simulink model "DemonstratorSimscape"  (R2020b)
settings: Solver=ode113  StartTime=0.0  StopTime=t_stop*0+20  FixedStep=1e-4
values from neighbouring files (symbols this model uses):
  brkD = 0    [main.m]
  brkI = 1e4    (= 10000)    [main.m]
  brkP = 1e5    (= 100000)    [main.m]
  d_drm = 0.5*d_drum    [main.m]
  d_shm = 0.4*d_sheave    [main.m]
  DeltaCable0 = 0    [main.m]
  Droop_scaling = 0    [main.m]
  eta_sh = 0.015    [main.m]
  filt_NUM = ones(1,200)*0.005    [main.m]
  g = 9.80665    [main.m]
  Iw = 0.5*(W.i + M.in*GB.r^2)    [main.m]
  Kp_mul = 0.3    [main.m]
  Lc0 = abs((T.ph-L.height-P.d-L.z0)*0.001)    [main.m]
  Ls1 = ((T.ph-0.5*W.pd)/1000)    [main.m]
  Ls2 = ((0.5*(T.s2+P.d)-2*P.d)/1000)    [main.m]
  M = 50e3    (= 50000)    [calcGrav.m]
  phi0_drm = -90    [main.m]
  phi0_shm = -90    [main.m]
  r_sheave = P.d*0.5    [main.m]
  s = tf('s')    [calcGrav.m]
  tau_brk = 0.001    [main.m]
  tau_em = 60e-3    (= 0.06)    [calcGrav.m]    (also in main.m)
  tau_m = tau_w/GB.r    [main.m]
  Tmax = 400e3    (= 400000)    [main.m]
  Tn_mul = 10    [main.m]
  x_drm = 0.7*r_drum    [main.m]
  x_shm = 0.7*r_sheave    [main.m]
  z0 = 0    [calcGrav.m]    (also in main.m = L.z0-P.d*0.5-P.d-P.d-L.height-T.h1-T.h2-32)
undefined symbols (not defined in the file or in its folder): C, CA, Controller_sampleTime, DiscIntNeverNeededParam, GB, L, P, Part, T, VFD_acceleration_model_factor, VFD_Adapt_factor_lower_p1458, VFD_Adapt_factor_upper_p1459, VFD_Curr_limit_var_p0641, VFD_Current_limit_p0640, VFD_Id_setp_total_r1624, VFD_Iq, VFD_Kp_n_basic_p1460, VFD_M, VFD_M_accel_T_smooth_p1517, VFD_M_lim_var_fixS_src_p1551, VFD_M_max_lower_p1521, VFD_M_max_lower_scal_p1525, VFD_M_max_up_mot_scal_p1524, VFD_M_max_upper_p1520, VFD_n_act_T_smooth_p1442, VFD_n_ctr_Kp_n_up_scal_p1461, VFD_n_ctr_Tn_n_up_sca_p1463, VFD_n_ctrl_adapt_Kp_lower_p1456, VFD_n_ctrl_adapt_Kp_upper_p1457, VFD_n_ctrl_Adpt_sig_Kp_p1455, VFD_n_ctrl_Kp_scal_p1466, VFD_n_ctrl_n_lower_p1464, VFD_n_ctrl_n_upper_p1465, VFD_n_ctrl_Tn_n_lower_p1462, VFD_n_limit_neg_p1086, VFD_n_limit_pos_p1083, VFD_n_limit_setp_p1063, VFD_n_max_p1082, VFD_n_set_filt_1_T_p1416, VFD_P_max_gen_p1531, VFD_P_max_mot_p1530, VFD_PU_I_outp_max_r0289, VFD_RFG_ramp_down_time_p1121, VFD_RFG_ramp_up_time_p1120, VFD_RFG_t_RD_scal_p1139, VFD_RFG_t_RU_scal_p1138, VSD, W, X, Y, Z
libraries: sm_lib x248, nesl_utility x128, simulink x49, pid_lib x4, cstblocks x2, simulink_extras x2
(part 8 of 10)

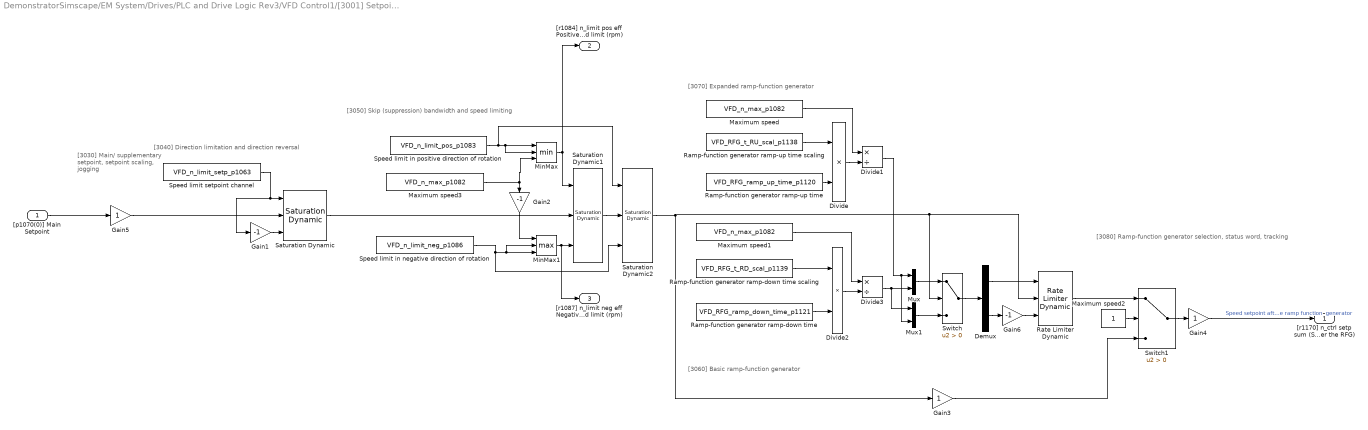
== system DemonstratorSimscape/EM System/Drives/PLC and Drive Logic Rev3/VFD Control1/[3001] Setpoint Channel  ==
  note: [3080] Ramp-function generator selection,
      | status word, tracking
  note: [3070] Expanded ramp-function generator
  note: [3040] Direction limitation and direction reversal
  note: [3050] Skip (suppression) bandwidth
      |  and speed limiting
  note: [3060] Basic ramp-function generator
  note: [3030] Main/
      | supplementary
      | setpoint,
      | setpoint
      | scaling,
      | jogging
  "[p1070(0)] Main Setpoint" : Inport
  Demux : Demux  Outputs=2
  Divide : Product  Inputs=**
  Divide1 : Product  Inputs=*/
  Divide2 : Product  Inputs=**
  Divide3 : Product  Inputs=*/
  Gain1 : Gain  Gain=-1
  Gain2 : Gain  Gain=-1
  Gain3 : Gain
  Gain4 : Gain
  Gain5 : Gain
  Gain6 : Gain  Gain=-1
  Maximum speed : Constant  Value=VFD_n_max_p1082
  Maximum speed1 : Constant  Value=VFD_n_max_p1082
  Maximum speed2 : Constant
  Maximum speed3 : Constant  Value=VFD_n_max_p1082
  MinMax : MinMax  Inputs=3
  MinMax1 : MinMax  Function=max  Inputs=3
  Mux : Mux  Inputs=2
  Mux1 : Mux  Inputs=2
  Ramp-function generator ramp-down time : Constant  Value=VFD_RFG_ramp_down_time_p1121
  Ramp-function generator ramp-down time scaling : Constant  Value=VFD_RFG_t_RD_scal_p1139  VectorParams1D=off
  "Ramp-function generator ramp-up time " : Constant  Value=VFD_RFG_ramp_up_time_p1120
  "Ramp-function generator ramp-up time scaling " : Constant  Value=VFD_RFG_t_RU_scal_p1138
  Rate Limiter Dynamic : simulink/Discontinuities/Rate Limiter Dynamic
  Saturation Dynamic : simulink/Discontinuities/Saturation Dynamic  OutMin=[]  OutMax=[]  OutDataTypeStr=Inherit: Same as second input  OutDataType=fixdt(1, 16)  OutScaling=2^-10  DoSatur=off
  Saturation Dynamic1 : simulink/Discontinuities/Saturation Dynamic  OutMin=[]  OutMax=[]  OutDataTypeStr=Inherit: Same as second input  OutDataType=fixdt(1, 16)  OutScaling=2^-10  DoSatur=off
  Saturation Dynamic2 : simulink/Discontinuities/Saturation Dynamic  OutMin=[]  OutMax=[]  OutDataTypeStr=Inherit: Same as second input  OutDataType=fixdt(1, 16)  OutScaling=2^-10  DoSatur=off
  "Speed limit in negative direction of rotation " : Constant  Value=VFD_n_limit_neg_p1086
  Speed limit in positive direction of rotation : Constant  Value=VFD_n_limit_pos_p1083
  Speed limit setpoint channel : Constant  Value=VFD_n_limit_setp_p1063
  Switch : Switch  Criteria=u2 > Threshold
  Switch1 : Switch  Criteria=u2 > Threshold
  "[r1170] n_ctrl setp sum (Speed setpoint after the RFG)" : Outport  VectorParamsAs1DForOutWhenUnconnected=off
  "[r1084] n_limit pos eff Positive Speed limit (rpm)" : Outport  Port=2  VectorParamsAs1DForOutWhenUnconnected=off
  "[r1087] n_limit neg eff Negative Speed limit (rpm)" : Outport  Port=3  VectorParamsAs1DForOutWhenUnconnected=off
  wires:
  Speed limit setpoint channel/1 -> Saturation Dynamic/1, Gain1/1
  Gain1/1 -> Saturation Dynamic/3
  "[p1070(0)] Main Setpoint"/1 -> Gain5/1
  MinMax1/1 -> "[r1087] n_limit neg eff Negative Speed limit (rpm)"/1, Saturation Dynamic1/3
  Saturation Dynamic/1 -> Saturation Dynamic1/2
  Speed limit in positive direction of rotation/1 -> Saturation Dynamic2/1, MinMax/2, MinMax/1
  "Speed limit in negative direction of rotation "/1 -> Saturation Dynamic2/3, MinMax1/2, MinMax1/3
  Maximum speed3/1 -> Gain2/1, MinMax/3
  MinMax/1 -> "[r1084] n_limit pos eff Positive Speed limit (rpm)"/1, Saturation Dynamic1/1
  Saturation Dynamic2/1 -> Gain3/1, Rate Limiter Dynamic/2, Switch/2
  Mux/1 -> Switch/1
  Maximum speed/1 -> Divide1/1
  Demux/2 -> Gain6/1
  Divide3/1 -> Mux1/1, Mux/2
  "Ramp-function generator ramp-up time scaling "/1 -> Divide/1
  Mux1/1 -> Switch/3
  Switch/1 -> Demux/1
  Divide1/1 -> Mux/1, Mux1/2
  "Ramp-function generator ramp-up time "/1 -> Divide/2
  Divide2/1 -> Divide3/2
  Maximum speed1/1 -> Divide3/1
  Ramp-function generator ramp-down time scaling/1 -> Divide2/1
  Ramp-function generator ramp-down time/1 -> Divide2/2
  Divide/1 -> Divide1/2
  Demux/1 -> Rate Limiter Dynamic/1
  Gain4/1 -> "[r1170] n_ctrl setp sum (Speed setpoint after the RFG)"/1  "Speed setpoint after  the ramp function  generator"
  Rate Limiter Dynamic/1 -> Switch1/1
  Switch1/1 -> Gain4/1
  Gain3/1 -> Switch1/3
  Maximum speed2/1 -> Switch1/2
  Gain5/1 -> Saturation Dynamic/2
  Gain6/1 -> Rate Limiter Dynamic/3
  Saturation Dynamic1/1 -> Saturation Dynamic2/2
  Gain2/1 -> MinMax1/1

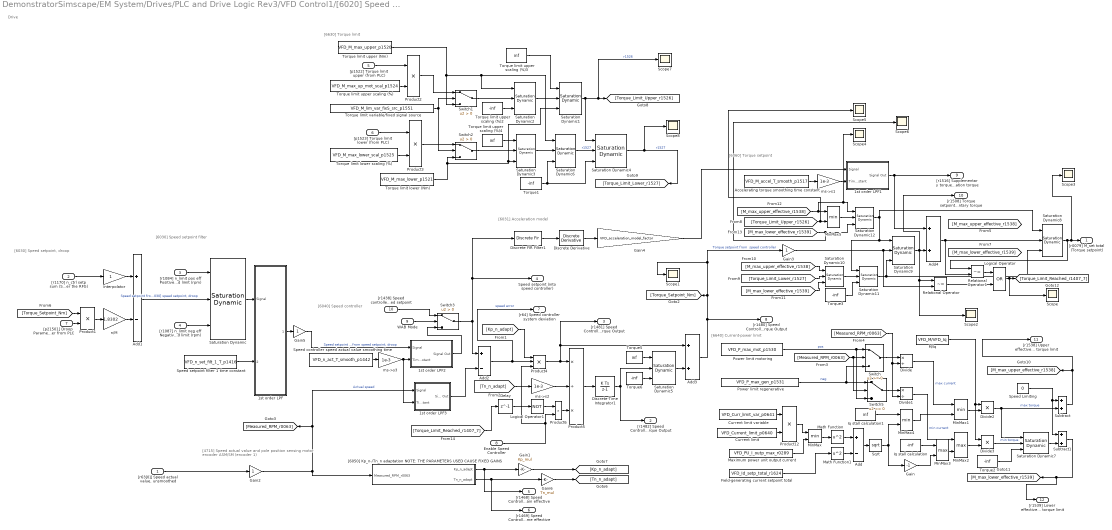
== system DemonstratorSimscape/EM System/Drives/PLC and Drive Logic Rev3/VFD Control1/[6020] Speed control and generation of the torque limits  ==
  note: [6030] Speed setpoint filter
  note: [6031] Acceleration model
  note: [4715] Speed actual value and pole position
      |  sensing motor encoder ASM/SM (encoder 1)
  note: [6630] Torque limit
  note: Drive
  note: [6030] Speed setpoint, droop
  note: [6040] Speed controller
  note: [6060] Torque setpoint
  note: [6640] Current-power limit
  "[r63[0]] Speed actual value, unsmoothed" : Inport
  "[r1170] n_ctrl setp sum (Speed setpoint after the RFG)" : Inport  Port=2
  "[r1084] n_limit pos eff Positive Speed limit (rpm)" : Inport  Port=3
  "[r1087] n_limit neg eff Negative Speed limit (rpm)" : Inport  Port=4
  "[p1522] Torque limit upper (from PLC)" : Inport  Port=5
  "[p1523] Torque limit lower (from PLC)" : Inport  Port=6
  "[p21501] Droop Parameter from PLC" : Inport  Port=7
  Enable Speed Controller : Inport  Port=8
  WAB Mode : Inport  Port=9
  "[r1438] Speed controller speed setpoint" : Inport  Port=10
  1st order LPF : Subsystem  mask{time_constant=0.1, Yo=0}
      mask prompts: time_constant "Time Constant (s)"; Yo "Initial Condition"
  1st order LPF1 : Subsystem  mask{time_constant=0.1, Yo=0}
      mask prompts: time_constant "Time Constant (s)"; Yo "Initial Condition"
  1st order LPF2 : Subsystem  mask{time_constant=0.1, Yo=0}
      mask prompts: time_constant "Time Constant (s)"; Yo "Initial Condition"
  1st order LPF3 : Subsystem  mask{time_constant=0.1, Yo=0}
      mask prompts: time_constant "Time Constant (s)"; Yo "Initial Condition"
  Accelerating torque smoothing time constant : Constant  Value=VFD_M_accel_T_smooth_p1517
  Add : Sum  Inputs=+-
  Add1 : Sum  Inputs=+-
  Add2 : Sum  Inputs=+-
  Add3 : Sum
  Add4 : Sum
  Current limit : Constant  Value=VFD_Current_limit_p0640
  Current limit variable : Constant  Value=VFD_Curr_limit_var_p0641
  Delay : Delay  DelayLength=1
  Discrete Derivative : simulink/Discrete/Discrete Derivative  gainval=1.0  ICPrevScaledInput=0.0  OutMin=[]  OutMax=[]  OutDataType=fixdt(1, 16)  OutScaling=2^-10  DoSatur=off
  Discrete FIR Filter1 : DiscreteFir  Coefficients=filt_NUM
  Discrete-Time Integrator1 : DiscreteIntegrator  InitialCondition=-tau_m  SampleTime=0.001  ICPrevOutput=DiscIntNeverNeededParam  ICPrevScaledInput=DiscIntNeverNeededParam
  Divide : Product  Inputs=*/
  Divide1 : Product  Inputs=*/
  Divide2 : Product  Inputs=**
  Divide3 : Product  Inputs=**
  Field-generating current setpoint total : Constant  Value=VFD_Id_setp_total_r1624
  Gain : Gain  Gain=-1
  Gain1 : Gain  Gain=Kp_mul
  Gain2 : Gain
  Gain3 : Gain
  Gain4 : Gain  Gain=VFD_acceleration_model_factor
  Gain5 : Gain
  Gain6 : Gain  Gain=Tn_mul
  Interpolator : Gain
  Iq stall calculation : Constant  Value=-inf
  Iq stall calculation1 : Constant  Value=inf
  Logical Operator : Logic  Operator=OR  AllPortsSameDT=off  OutDataTypeStr=boolean
  Logical Operator1 : Logic  Operator=NOT  AllPortsSameDT=off  OutDataTypeStr=boolean
  M/Iq : Constant  Value=VFD_M/VFD_Iq
  Math Function : Math  Operator=square  SaturateOnIntegerOverflow=on
  Math Function1 : Math  Operator=square  SaturateOnIntegerOverflow=on
  Maximum power unit output current : Constant  Value=VFD_PU_I_outp_max_r0289
  MinMax{,1,4..5} (4 alike) : MinMax  Inputs=2
  MinMax2 : MinMax  Function=max  Inputs=2
  MinMax3 : MinMax  Function=max  Inputs=2
  Power limit motoring : Constant  Value=VFD_P_max_mot_p1530
  Power limit regenerative : Constant  Value=VFD_P_max_gen_p1531
  Product1 : Product  Inputs=**
  Product12 : Product
  Product2 : Product
  Product3 : Product
  Product4 : Product  Inputs=3
  Product5 : Product  Inputs=*/*
  Product6 : Product  Inputs=**
  Relational Operator : RelationalOperator  Operator=~=  OutDataTypeStr=boolean  RndMeth=Simplest
  Relational Operator1 : RelationalOperator  Operator=~=  OutDataTypeStr=boolean  RndMeth=Simplest
  Saturation Dynamic{,1..12} (13 alike) : simulink/Discontinuities/Saturation Dynamic  OutMin=[]  OutMax=[]  OutDataTypeStr=Inherit: Same as second input  OutDataType=fixdt(1, 16)  OutScaling=2^-10  DoSatur=off
  Scope{,1..8} (9 alike) : Scope
  Speed Limiting : Constant  Value=0
  Speed controller speed actual value smoothing time : Constant  Value=VFD_n_act_T_smooth_p1442
  "Speed setpoint filter 1 time constant " : Constant  Value=VFD_n_set_filt_1_T_p1416
  Sqrt : Sqrt  SaturateOnIntegerOverflow=on
  Subtract : Sum
  Subtract1 : Sum
  Switch : Switch
  Switch1 : Switch  Criteria=u2 > Threshold
  Switch2 : Switch  Criteria=u2 > Threshold
  Switch3 : Switch  Criteria=u2 > Threshold
  Switch5 : Switch
  Torque limit lower (Nm) : Constant  Value=VFD_M_max_lower_p1521
  Torque limit lower scaling (%) : Constant  Value=VFD_M_max_lower_scal_p1525
  Torque limit upper (Nm) : Constant  Value=VFD_M_max_upper_p1520
  Torque limit upper scaling (%) : Constant  Value=VFD_M_max_up_mot_scal_p1524
  Torque limit upper scaling (%)2 : Constant  Value=-inf
  Torque limit upper scaling (%)3 : Constant  Value=inf
  Torque limit upper scaling (%)4 : Constant  Value=inf
  Torque limit variable/fixed signal source : Constant  Value=VFD_M_lim_var_fixS_src_p1551
  Torque{1..3,6} (4 alike) : Constant  Value=-inf
  Torque5 : Constant  Value=inf
  "[6050] Kp_n-/Tn_n adaptation NOTE: THE PARAMETERS USED CAUSE FIXED GAINS" : Subsystem
  ms->s1 : Gain  Gain=1e-3
  ms->s2 : Gain  Gain=1e-3
  ms->s3 : Gain  Gain=1e-3
  n/M : Gain  Gain=1.8302
  "[r0079] M_set total (Torque setpoint)" : Outport  VectorParamsAs1DForOutWhenUnconnected=off
  "[r1482] Speed Controller I torque Output" : Outport  Port=2  VectorParamsAs1DForOutWhenUnconnected=off
  "[r1481] Speed Controller P torque Output" : Outport  Port=3  VectorParamsAs1DForOutWhenUnconnected=off
  Speed setpoint (into speed controller) : Outport  Port=4  VectorParamsAs1DForOutWhenUnconnected=off
  "[r1468] Speed Controller P-gain effective" : Outport  Port=5  VectorParamsAs1DForOutWhenUnconnected=off
  "[r1469] Speed Controller integral time effective" : Outport  Port=6  VectorParamsAs1DForOutWhenUnconnected=off
  "[r64] Speed controller system deviation" : Outport  Port=7  VectorParamsAs1DForOutWhenUnconnected=off
  "[r1480] Speed Controller PI torque Output" : Outport  Port=8  VectorParamsAs1DForOutWhenUnconnected=off
  "[r1516] Supplementary torque and acceleration torque " : Outport  Port=9  VectorParamsAs1DForOutWhenUnconnected=off
  "[r1508] Torque setpoint before supplementary torque" : Outport  Port=10  VectorParamsAs1DForOutWhenUnconnected=off
  "[r1538] Upper effective torque limit" : Outport  Port=11  VectorParamsAs1DForOutWhenUnconnected=off
  "[r1539] Lower effective torque limit" : Outport  Port=12  VectorParamsAs1DForOutWhenUnconnected=off
  wires:
  Discrete Derivative/1 -> Gain4/1
  Switch3/1 -> Speed setpoint (into speed controller)/1, Discrete FIR Filter1/1, Add2/1
  "[6050] Kp_n-/Tn_n adaptation NOTE: THE PARAMETERS USED CAUSE FIXED GAINS"/2(Tn_n_adapt) -> Gain6/1, "[r1469] Speed Controller integral time effective"/1
  "[r1438] Speed controller speed setpoint"/1 -> Switch3/1
  1st order LPF2/1(Signal Out) -> Switch3/3
  WAB Mode/1 -> Switch3/2
  "[r63[0]] Speed actual value, unsmoothed"/1 -> Gain2/1
  Saturation Dynamic/1 -> 1st order LPF/1(Signal)
  "[r1084] n_limit pos eff Positive Speed limit (rpm)"/1 -> Saturation Dynamic/1
  "[r1087] n_limit neg eff Negative Speed limit (rpm)"/1 -> Saturation Dynamic/3
  "Speed setpoint filter 1 time constant "/1 -> 1st order LPF/2(Time Constant)
  Product2/1 -> Switch1/1
  Switch1/1 -> Saturation Dynamic2/2
  Switch2/1 -> Saturation Dynamic3/2
  Saturation Dynamic3/1 -> Saturation Dynamic6/2
  Saturation Dynamic1/1 -> Scope7/1, [Torque_Limit_Upper_r1526], Saturation Dynamic4/1  "r1526"
  Torque1/1 -> Saturation Dynamic4/3, Saturation Dynamic6/3
  Torque limit upper (Nm)/1 -> Switch1/3, Saturation Dynamic6/1, Saturation Dynamic2/1
  "[p1522] Torque limit upper (from PLC)"/1 -> Product2/1
  Torque limit upper scaling (%)/1 -> Product2/2
  Torque limit lower (Nm)/1 -> Switch2/3, Saturation Dynamic3/3, Saturation Dynamic1/3
  Torque limit lower scaling (%)/1 -> Product3/2
  Saturation Dynamic4/1 -> Scope8/1, [Torque_Limit_Lower_r1527]  "r1527"
  [Torque_Setpoint_Nm] -> Product1/1
  Discrete-Time Integrator1/1 -> "[r1482] Speed Controller I torque Output"/1, Saturation Dynamic5/2
  Product1/1 -> n/M/1
  [Tn_n_adapt] -> ms->s2/1
  Saturation Dynamic5/1 -> Add3/2
  Interpolator/1 -> Add1/1
  Product4/1 -> Product5/1, Add3/1, "[r1481] Speed Controller P torque Output"/1
  n/M/1 -> Add1/2
  [Kp_n_adapt] -> Product4/1
  Torque6/1 -> Saturation Dynamic5/3
  Add2/1 -> Product4/2, "[r64] Speed controller system deviation"/1  "speed error"
  Torque5/1 -> Saturation Dynamic5/1
  Add3/1 -> [Torque_Setpoint_Nm], Scope1/1, Gain3/1, "[r1480] Speed Controller PI torque Output"/1  "Torque setpoint from  speed controller"
  Product5/1 -> Discrete-Time Integrator1/1
  ms->s2/1 -> Product5/2
  1st order LPF/1(Signal Out) -> Gain5/1
  Speed controller speed actual value smoothing time/1 -> ms->s3/1
  Gain5/1 -> 1st order LPF2/1(Signal)  "Speed setpoint from speed setpoint, droop"
  Gain2/1 -> "[6050] Kp_n-/Tn_n adaptation NOTE: THE PARAMETERS USED CAUSE FIXED GAINS"/1(Measured_RPM_r0063), [Measured_RPM_r0063], 1st order LPF3/1(Signal)  "Actual speed"
  ms->s3/1 -> 1st order LPF2/2(Time Constant), 1st order LPF3/2(Time Constant)
  1st order LPF3/1(Signal Out) -> Add2/2
  Saturation Dynamic8/1 -> Relational Operator1/1, Scope3/1, "[r0079] M_set total (Torque setpoint)"/1
  Torque limit variable/fixed signal source/1 -> Switch1/2, Switch2/2
  Torque limit upper scaling (%)2/1 -> Saturation Dynamic2/3
  Saturation Dynamic2/1 -> Saturation Dynamic1/2
  Torque limit upper scaling (%)3/1 -> Saturation Dynamic1/1
  "[p1523] Torque limit lower (from PLC)"/1 -> Product3/1
  Product3/1 -> Switch2/1
  Torque limit upper scaling (%)4/1 -> Saturation Dynamic3/1
  Saturation Dynamic6/1 -> Saturation Dynamic4/2  "r1527"
  Power limit regenerative/1 -> Switch5/1, Switch/3  "neg"
  Power limit motoring/1 -> Switch5/3, Switch/1  "pos"
  [Measured_RPM_r0063] -> Switch5/2, Switch/2
  Switch/1 -> Divide/1
  Switch5/1 -> Divide1/1
  [Measured_RPM_r0063] -> Divide1/2, Divide/2
  Current limit variable/1 -> Product12/1
  Current limit/1 -> Product12/2
  Product12/1 -> MinMax/1
  Maximum power unit output current/1 -> MinMax/2
  MinMax/1 -> Math Function/1
  Field-generating current setpoint total/1 -> Math Function1/1
  Math Function/1 -> Add/1
  Math Function1/1 -> Add/2
  Add/1 -> Sqrt/1
  Sqrt/1 -> MinMax4/2, Gain/1
  Divide/1 -> MinMax1/1  "max current"
  Divide1/1 -> MinMax2/1  "min current"
  Gain/1 -> MinMax3/2
  MinMax1/1 -> Divide2/2
  MinMax2/1 -> Divide3/2
  M/Iq/1 -> Divide2/1, Divide3/1
  Divide3/1 -> Saturation Dynamic7/2  "min torque"
  Torque2/1 -> Saturation Dynamic7/3
  Divide2/1 -> Subtract/2, Saturation Dynamic7/1  "max torque"
  Speed Limiting/1 -> Subtract/1, Subtract1/1
  Saturation Dynamic7/1 -> Subtract1/2
  Subtract/1 -> [M_max_upper_effective_r1538], "[r1538] Upper effective torque limit"/1
  Subtract1/1 -> [M_max_lower_effective_r1539], "[r1539] Lower effective torque limit"/1
  MinMax3/1 -> MinMax2/2
  Iq stall calculation/1 -> MinMax3/1
  MinMax4/1 -> MinMax1/2
  Iq stall calculation1/1 -> MinMax4/1
  Add4/1 -> Relational Operator1/2, Saturation Dynamic8/2
  1st order LPF1/1(Signal Out) -> "[r1516] Supplementary torque and acceleration torque "/1, Add4/1
  Gain3/1 -> Saturation Dynamic9/2, Relational Operator/2
  Saturation Dynamic9/1 -> Add4/2, Scope2/1, Relational Operator/1, "[r1508] Torque setpoint before supplementary torque"/1
  [Torque_Limit_Lower_r1527] -> Saturation Dynamic10/2
  Saturation Dynamic11/1 -> Saturation Dynamic9/3, Saturation Dynamic8/3
  [M_max_upper_effective_r1538] -> Saturation Dynamic10/1
  [M_max_lower_effective_r1539] -> Saturation Dynamic10/3
  Torque3/1 -> Saturation Dynamic11/3
  Saturation Dynamic10/1 -> Saturation Dynamic11/2
  [Torque_Limit_Upper_r1526] -> Scope5/1, MinMax5/2
  [M_max_upper_effective_r1538] -> MinMax5/1, Scope4/1, Saturation Dynamic12/1
  Saturation Dynamic12/1 -> Saturation Dynamic9/1, Saturation Dynamic11/1, Saturation Dynamic8/1
  MinMax5/1 -> Saturation Dynamic12/2
  [M_max_lower_effective_r1539] -> Scope6/1, Saturation Dynamic12/3
  Relational Operator/1 -> Logical Operator/2
  Relational Operator1/1 -> Logical Operator/1
  Logical Operator/1 -> Scope/1, [Torque_Limit_Reached_r1407_7]
  [Torque_Limit_Reached_r1407_7] -> Delay/1
  Product6/1 -> Product5/3
  Accelerating torque smoothing time constant/1 -> ms->s1/1
  ms->s1/1 -> 1st order LPF1/2(Time Constant)
  Gain4/1 -> 1st order LPF1/1(Signal)
  Delay/1 -> Logical Operator1/1
  Add1/1 -> Saturation Dynamic/2  "Speed setpoint from  [6030] speed setpoint, droop"
  "[r1170] n_ctrl setp sum (Speed setpoint after the RFG)"/1 -> Interpolator/1
  "[6050] Kp_n-/Tn_n adaptation NOTE: THE PARAMETERS USED CAUSE FIXED GAINS"/1(Kp_n_adapt) -> Gain1/1, "[r1468] Speed Controller P-gain effective"/1
  "[p21501] Droop Parameter from PLC"/1 -> Product1/2
  Logical Operator1/1 -> Product6/1
  Enable Speed Controller/1 -> Product4/3, Product6/2
  Gain1/1 -> [Kp_n_adapt]
  Gain6/1 -> [Tn_n_adapt]
  Discrete FIR Filter1/1 -> Discrete Derivative/1

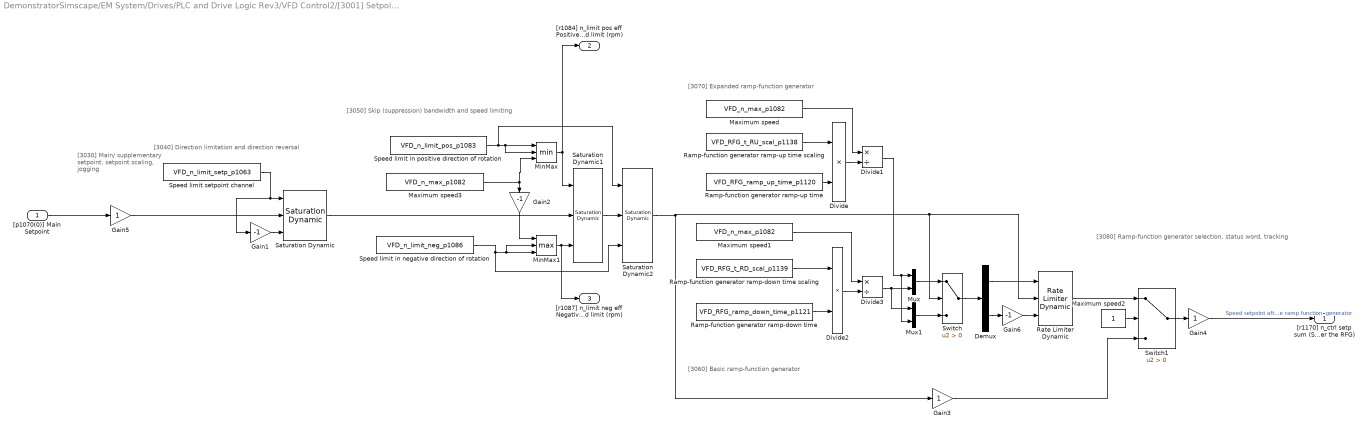
== system DemonstratorSimscape/EM System/Drives/PLC and Drive Logic Rev3/VFD Control2/[3001] Setpoint Channel  ==
  note: [3080] Ramp-function generator selection,
      | status word, tracking
  note: [3070] Expanded ramp-function generator
  note: [3040] Direction limitation and direction reversal
  note: [3050] Skip (suppression) bandwidth
      |  and speed limiting
  note: [3060] Basic ramp-function generator
  note: [3030] Main/
      | supplementary
      | setpoint,
      | setpoint
      | scaling,
      | jogging
  "[p1070(0)] Main Setpoint" : Inport
  Demux : Demux  Outputs=2
  Divide : Product  Inputs=**
  Divide1 : Product  Inputs=*/
  Divide2 : Product  Inputs=**
  Divide3 : Product  Inputs=*/
  Gain1 : Gain  Gain=-1
  Gain2 : Gain  Gain=-1
  Gain3 : Gain
  Gain4 : Gain
  Gain5 : Gain
  Gain6 : Gain  Gain=-1
  Maximum speed : Constant  Value=VFD_n_max_p1082
  Maximum speed1 : Constant  Value=VFD_n_max_p1082
  Maximum speed2 : Constant
  Maximum speed3 : Constant  Value=VFD_n_max_p1082
  MinMax : MinMax  Inputs=3
  MinMax1 : MinMax  Function=max  Inputs=3
  Mux : Mux  Inputs=2
  Mux1 : Mux  Inputs=2
  Ramp-function generator ramp-down time : Constant  Value=VFD_RFG_ramp_down_time_p1121
  Ramp-function generator ramp-down time scaling : Constant  Value=VFD_RFG_t_RD_scal_p1139  VectorParams1D=off
  "Ramp-function generator ramp-up time " : Constant  Value=VFD_RFG_ramp_up_time_p1120
  "Ramp-function generator ramp-up time scaling " : Constant  Value=VFD_RFG_t_RU_scal_p1138
  Rate Limiter Dynamic : simulink/Discontinuities/Rate Limiter Dynamic
  Saturation Dynamic : simulink/Discontinuities/Saturation Dynamic  OutMin=[]  OutMax=[]  OutDataTypeStr=Inherit: Same as second input  OutDataType=fixdt(1, 16)  OutScaling=2^-10  DoSatur=off
  Saturation Dynamic1 : simulink/Discontinuities/Saturation Dynamic  OutMin=[]  OutMax=[]  OutDataTypeStr=Inherit: Same as second input  OutDataType=fixdt(1, 16)  OutScaling=2^-10  DoSatur=off
  Saturation Dynamic2 : simulink/Discontinuities/Saturation Dynamic  OutMin=[]  OutMax=[]  OutDataTypeStr=Inherit: Same as second input  OutDataType=fixdt(1, 16)  OutScaling=2^-10  DoSatur=off
  "Speed limit in negative direction of rotation " : Constant  Value=VFD_n_limit_neg_p1086
  Speed limit in positive direction of rotation : Constant  Value=VFD_n_limit_pos_p1083
  Speed limit setpoint channel : Constant  Value=VFD_n_limit_setp_p1063
  Switch : Switch  Criteria=u2 > Threshold
  Switch1 : Switch  Criteria=u2 > Threshold
  "[r1170] n_ctrl setp sum (Speed setpoint after the RFG)" : Outport  VectorParamsAs1DForOutWhenUnconnected=off
  "[r1084] n_limit pos eff Positive Speed limit (rpm)" : Outport  Port=2  VectorParamsAs1DForOutWhenUnconnected=off
  "[r1087] n_limit neg eff Negative Speed limit (rpm)" : Outport  Port=3  VectorParamsAs1DForOutWhenUnconnected=off
  wires:
  Speed limit setpoint channel/1 -> Saturation Dynamic/1, Gain1/1
  Gain1/1 -> Saturation Dynamic/3
  "[p1070(0)] Main Setpoint"/1 -> Gain5/1
  MinMax1/1 -> "[r1087] n_limit neg eff Negative Speed limit (rpm)"/1, Saturation Dynamic1/3
  Saturation Dynamic/1 -> Saturation Dynamic1/2
  Speed limit in positive direction of rotation/1 -> Saturation Dynamic2/1, MinMax/2, MinMax/1
  "Speed limit in negative direction of rotation "/1 -> Saturation Dynamic2/3, MinMax1/2, MinMax1/3
  Maximum speed3/1 -> Gain2/1, MinMax/3
  MinMax/1 -> "[r1084] n_limit pos eff Positive Speed limit (rpm)"/1, Saturation Dynamic1/1
  Saturation Dynamic2/1 -> Gain3/1, Rate Limiter Dynamic/2, Switch/2
  Mux/1 -> Switch/1
  Maximum speed/1 -> Divide1/1
  Demux/2 -> Gain6/1
  Divide3/1 -> Mux1/1, Mux/2
  "Ramp-function generator ramp-up time scaling "/1 -> Divide/1
  Mux1/1 -> Switch/3
  Switch/1 -> Demux/1
  Divide1/1 -> Mux/1, Mux1/2
  "Ramp-function generator ramp-up time "/1 -> Divide/2
  Divide2/1 -> Divide3/2
  Maximum speed1/1 -> Divide3/1
  Ramp-function generator ramp-down time scaling/1 -> Divide2/1
  Ramp-function generator ramp-down time/1 -> Divide2/2
  Divide/1 -> Divide1/2
  Demux/1 -> Rate Limiter Dynamic/1
  Gain4/1 -> "[r1170] n_ctrl setp sum (Speed setpoint after the RFG)"/1  "Speed setpoint after  the ramp function  generator"
  Rate Limiter Dynamic/1 -> Switch1/1
  Switch1/1 -> Gain4/1
  Gain3/1 -> Switch1/3
  Maximum speed2/1 -> Switch1/2
  Gain5/1 -> Saturation Dynamic/2
  Gain6/1 -> Rate Limiter Dynamic/3
  Saturation Dynamic1/1 -> Saturation Dynamic2/2
  Gain2/1 -> MinMax1/1

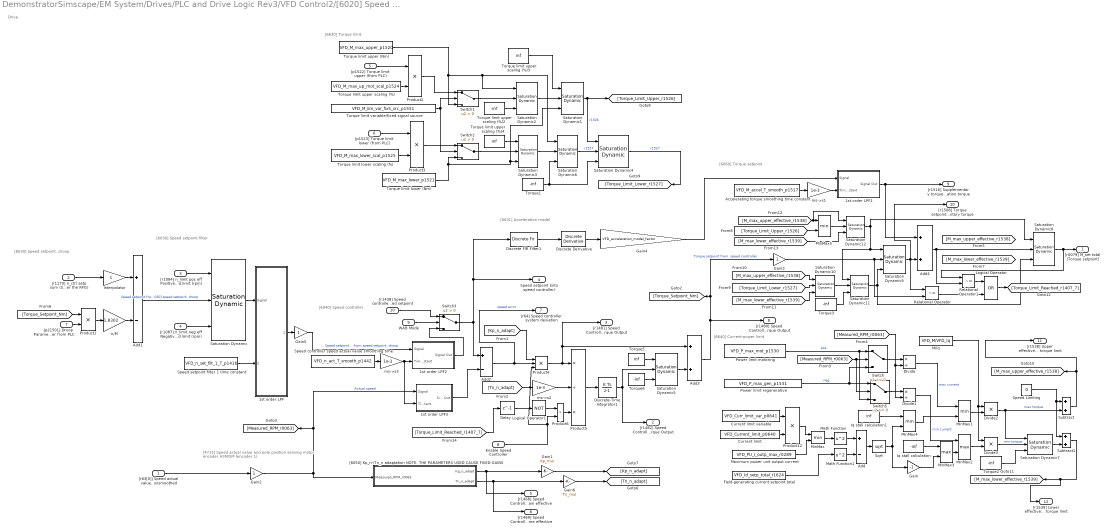
== system DemonstratorSimscape/EM System/Drives/PLC and Drive Logic Rev3/VFD Control2/[6020] Speed control and generation of the torque limits  ==
  note: [6030] Speed setpoint filter
  note: [6031] Acceleration model
  note: [4715] Speed actual value and pole position
      |  sensing motor encoder ASM/SM (encoder 1)
  note: [6630] Torque limit
  note: Drive
  note: [6030] Speed setpoint, droop
  note: [6040] Speed controller
  note: [6060] Torque setpoint
  note: [6640] Current-power limit
  "[r63[0]] Speed actual value, unsmoothed" : Inport
  "[r1170] n_ctrl setp sum (Speed setpoint after the RFG)" : Inport  Port=2
  "[r1084] n_limit pos eff Positive Speed limit (rpm)" : Inport  Port=3
  "[r1087] n_limit neg eff Negative Speed limit (rpm)" : Inport  Port=4
  "[p1522] Torque limit upper (from PLC)" : Inport  Port=5
  "[p1523] Torque limit lower (from PLC)" : Inport  Port=6
  "[p21501] Droop Parameter from PLC" : Inport  Port=7
  Enable Speed Controller : Inport  Port=8
  WAB Mode : Inport  Port=9
  "[r1438] Speed controller speed setpoint" : Inport  Port=10
  1st order LPF : Subsystem  mask{time_constant=0.1, Yo=0}
      mask prompts: time_constant "Time Constant (s)"; Yo "Initial Condition"
  1st order LPF1 : Subsystem  mask{time_constant=0.1, Yo=0}
      mask prompts: time_constant "Time Constant (s)"; Yo "Initial Condition"
  1st order LPF2 : Subsystem  mask{time_constant=0.1, Yo=0}
      mask prompts: time_constant "Time Constant (s)"; Yo "Initial Condition"
  1st order LPF3 : Subsystem  mask{time_constant=0.1, Yo=0}
      mask prompts: time_constant "Time Constant (s)"; Yo "Initial Condition"
  Accelerating torque smoothing time constant : Constant  Value=VFD_M_accel_T_smooth_p1517
  Add : Sum  Inputs=+-
  Add1 : Sum  Inputs=+-
  Add2 : Sum  Inputs=+-
  Add3 : Sum
  Add4 : Sum
  Current limit : Constant  Value=VFD_Current_limit_p0640
  Current limit variable : Constant  Value=VFD_Curr_limit_var_p0641
  Delay : Delay  DelayLength=1
  Discrete Derivative : simulink/Discrete/Discrete Derivative  gainval=1.0  ICPrevScaledInput=0.0  OutMin=[]  OutMax=[]  OutDataType=fixdt(1, 16)  OutScaling=2^-10  DoSatur=off
  Discrete FIR Filter1 : DiscreteFir  Coefficients=filt_NUM
  Discrete-Time Integrator1 : DiscreteIntegrator  InitialCondition=tau_m  SampleTime=0.001  ICPrevOutput=DiscIntNeverNeededParam  ICPrevScaledInput=DiscIntNeverNeededParam
  Divide : Product  Inputs=*/
  Divide1 : Product  Inputs=*/
  Divide2 : Product  Inputs=**
  Divide3 : Product  Inputs=**
  Field-generating current setpoint total : Constant  Value=VFD_Id_setp_total_r1624
  Gain : Gain  Gain=-1
  Gain1 : Gain  Gain=Kp_mul
  Gain2 : Gain
  Gain3 : Gain
  Gain4 : Gain  Gain=VFD_acceleration_model_factor
  Gain5 : Gain
  Gain6 : Gain  Gain=Tn_mul
  Interpolator : Gain
  Iq stall calculation : Constant  Value=-inf
  Iq stall calculation1 : Constant  Value=inf
  Logical Operator : Logic  Operator=OR  AllPortsSameDT=off  OutDataTypeStr=boolean
  Logical Operator1 : Logic  Operator=NOT  AllPortsSameDT=off  OutDataTypeStr=boolean
  M/Iq : Constant  Value=VFD_M/VFD_Iq
  Math Function : Math  Operator=square  SaturateOnIntegerOverflow=on
  Math Function1 : Math  Operator=square  SaturateOnIntegerOverflow=on
  Maximum power unit output current : Constant  Value=VFD_PU_I_outp_max_r0289
  MinMax{,1,4..5} (4 alike) : MinMax  Inputs=2
  MinMax2 : MinMax  Function=max  Inputs=2
  MinMax3 : MinMax  Function=max  Inputs=2
  Power limit motoring : Constant  Value=VFD_P_max_mot_p1530
  Power limit regenerative : Constant  Value=VFD_P_max_gen_p1531
  Product1 : Product  Inputs=**
  Product12 : Product
  Product2 : Product
  Product3 : Product
  Product4 : Product  Inputs=3
  Product5 : Product  Inputs=*/*
  Product6 : Product  Inputs=**
  Relational Operator : RelationalOperator  Operator=~=  OutDataTypeStr=boolean  RndMeth=Simplest
  Relational Operator1 : RelationalOperator  Operator=~=  OutDataTypeStr=boolean  RndMeth=Simplest
  Saturation Dynamic{,1..12} (13 alike) : simulink/Discontinuities/Saturation Dynamic  OutMin=[]  OutMax=[]  OutDataTypeStr=Inherit: Same as second input  OutDataType=fixdt(1, 16)  OutScaling=2^-10  DoSatur=off
  Speed Limiting : Constant  Value=0
  Speed controller speed actual value smoothing time : Constant  Value=VFD_n_act_T_smooth_p1442
  "Speed setpoint filter 1 time constant " : Constant  Value=VFD_n_set_filt_1_T_p1416
  Sqrt : Sqrt  SaturateOnIntegerOverflow=on
  Subtract : Sum
  Subtract1 : Sum
  Switch : Switch
  Switch1 : Switch  Criteria=u2 > Threshold
  Switch2 : Switch  Criteria=u2 > Threshold
  Switch3 : Switch  Criteria=u2 > Threshold
  Switch5 : Switch
  Torque limit lower (Nm) : Constant  Value=VFD_M_max_lower_p1521
  Torque limit lower scaling (%) : Constant  Value=VFD_M_max_lower_scal_p1525
  Torque limit upper (Nm) : Constant  Value=VFD_M_max_upper_p1520
  Torque limit upper scaling (%) : Constant  Value=VFD_M_max_up_mot_scal_p1524
  Torque limit upper scaling (%)2 : Constant  Value=-inf
  Torque limit upper scaling (%)3 : Constant  Value=inf
  Torque limit upper scaling (%)4 : Constant  Value=inf
  Torque limit variable/fixed signal source : Constant  Value=VFD_M_lim_var_fixS_src_p1551
  Torque{1..3,6} (4 alike) : Constant  Value=-inf
  Torque5 : Constant  Value=inf
  "[6050] Kp_n-/Tn_n adaptation NOTE: THE PARAMETERS USED CAUSE FIXED GAINS" : Subsystem
  ms->s1 : Gain  Gain=1e-3
  ms->s2 : Gain  Gain=1e-3
  ms->s3 : Gain  Gain=1e-3
  n/M : Gain  Gain=1.8302
  "[r0079] M_set total (Torque setpoint)" : Outport  VectorParamsAs1DForOutWhenUnconnected=off
  "[r1482] Speed Controller I torque Output" : Outport  Port=2  VectorParamsAs1DForOutWhenUnconnected=off
  "[r1481] Speed Controller P torque Output" : Outport  Port=3  VectorParamsAs1DForOutWhenUnconnected=off
  Speed setpoint (into speed controller) : Outport  Port=4  VectorParamsAs1DForOutWhenUnconnected=off
  "[r1468] Speed Controller P-gain effective" : Outport  Port=5  VectorParamsAs1DForOutWhenUnconnected=off
  "[r1469] Speed Controller integral time effective" : Outport  Port=6  VectorParamsAs1DForOutWhenUnconnected=off
  "[r64] Speed controller system deviation" : Outport  Port=7  VectorParamsAs1DForOutWhenUnconnected=off
  "[r1480] Speed Controller PI torque Output" : Outport  Port=8  VectorParamsAs1DForOutWhenUnconnected=off
  "[r1516] Supplementary torque and acceleration torque " : Outport  Port=9  VectorParamsAs1DForOutWhenUnconnected=off
  "[r1508] Torque setpoint before supplementary torque" : Outport  Port=10  VectorParamsAs1DForOutWhenUnconnected=off
  "[r1538] Upper effective torque limit" : Outport  Port=11  VectorParamsAs1DForOutWhenUnconnected=off
  "[r1539] Lower effective torque limit" : Outport  Port=12  VectorParamsAs1DForOutWhenUnconnected=off
  wires:
  Discrete Derivative/1 -> Gain4/1
  Switch3/1 -> Speed setpoint (into speed controller)/1, Discrete FIR Filter1/1, Add2/1
  "[6050] Kp_n-/Tn_n adaptation NOTE: THE PARAMETERS USED CAUSE FIXED GAINS"/2(Tn_n_adapt) -> Gain6/1, "[r1469] Speed Controller integral time effective"/1
  "[r1438] Speed controller speed setpoint"/1 -> Switch3/1
  1st order LPF2/1(Signal Out) -> Switch3/3
  WAB Mode/1 -> Switch3/2
  "[r63[0]] Speed actual value, unsmoothed"/1 -> Gain2/1
  Saturation Dynamic/1 -> 1st order LPF/1(Signal)
  "[r1084] n_limit pos eff Positive Speed limit (rpm)"/1 -> Saturation Dynamic/1
  "[r1087] n_limit neg eff Negative Speed limit (rpm)"/1 -> Saturation Dynamic/3
  "Speed setpoint filter 1 time constant "/1 -> 1st order LPF/2(Time Constant)
  Product2/1 -> Switch1/1
  Switch1/1 -> Saturation Dynamic2/2
  Switch2/1 -> Saturation Dynamic3/2
  Saturation Dynamic3/1 -> Saturation Dynamic6/2
  Saturation Dynamic1/1 -> [Torque_Limit_Upper_r1526], Saturation Dynamic4/1  "r1526"
  Torque1/1 -> Saturation Dynamic4/3, Saturation Dynamic6/3
  Torque limit upper (Nm)/1 -> Switch1/3, Saturation Dynamic6/1, Saturation Dynamic2/1
  "[p1522] Torque limit upper (from PLC)"/1 -> Product2/1
  Torque limit upper scaling (%)/1 -> Product2/2
  Torque limit lower (Nm)/1 -> Switch2/3, Saturation Dynamic3/3, Saturation Dynamic1/3
  Torque limit lower scaling (%)/1 -> Product3/2
  Saturation Dynamic4/1 -> [Torque_Limit_Lower_r1527]  "r1527"
  [Torque_Setpoint_Nm] -> Product1/1
  Discrete-Time Integrator1/1 -> "[r1482] Speed Controller I torque Output"/1, Saturation Dynamic5/2
  Product1/1 -> n/M/1
  [Tn_n_adapt] -> ms->s2/1
  Saturation Dynamic5/1 -> Add3/2
  Interpolator/1 -> Add1/1
  Product4/1 -> Product5/1, Add3/1, "[r1481] Speed Controller P torque Output"/1
  n/M/1 -> Add1/2
  [Kp_n_adapt] -> Product4/1
  Torque6/1 -> Saturation Dynamic5/3
  Add2/1 -> Product4/2, "[r64] Speed controller system deviation"/1  "speed error"
  Torque5/1 -> Saturation Dynamic5/1
  Add3/1 -> [Torque_Setpoint_Nm], Gain3/1, "[r1480] Speed Controller PI torque Output"/1  "Torque setpoint from  speed controller"
  Product5/1 -> Discrete-Time Integrator1/1
  ms->s2/1 -> Product5/2
  1st order LPF/1(Signal Out) -> Gain5/1
  Speed controller speed actual value smoothing time/1 -> ms->s3/1
  Gain5/1 -> 1st order LPF2/1(Signal)  "Speed setpoint from speed setpoint, droop"
  Gain2/1 -> "[6050] Kp_n-/Tn_n adaptation NOTE: THE PARAMETERS USED CAUSE FIXED GAINS"/1(Measured_RPM_r0063), [Measured_RPM_r0063], 1st order LPF3/1(Signal)  "Actual speed"
  ms->s3/1 -> 1st order LPF2/2(Time Constant), 1st order LPF3/2(Time Constant)
  1st order LPF3/1(Signal Out) -> Add2/2
  Saturation Dynamic8/1 -> Relational Operator1/1, "[r0079] M_set total (Torque setpoint)"/1
  Torque limit variable/fixed signal source/1 -> Switch1/2, Switch2/2
  Torque limit upper scaling (%)2/1 -> Saturation Dynamic2/3
  Saturation Dynamic2/1 -> Saturation Dynamic1/2
  Torque limit upper scaling (%)3/1 -> Saturation Dynamic1/1
  "[p1523] Torque limit lower (from PLC)"/1 -> Product3/1
  Product3/1 -> Switch2/1
  Torque limit upper scaling (%)4/1 -> Saturation Dynamic3/1
  Saturation Dynamic6/1 -> Saturation Dynamic4/2  "r1527"
  Power limit regenerative/1 -> Switch5/1, Switch/3  "neg"
  Power limit motoring/1 -> Switch5/3, Switch/1  "pos"
  [Measured_RPM_r0063] -> Switch5/2, Switch/2
  Switch/1 -> Divide/1
  Switch5/1 -> Divide1/1
  [Measured_RPM_r0063] -> Divide1/2, Divide/2
  Current limit variable/1 -> Product12/1
  Current limit/1 -> Product12/2
  Product12/1 -> MinMax/1
  Maximum power unit output current/1 -> MinMax/2
  MinMax/1 -> Math Function/1
  Field-generating current setpoint total/1 -> Math Function1/1
  Math Function/1 -> Add/1
  Math Function1/1 -> Add/2
  Add/1 -> Sqrt/1
  Sqrt/1 -> MinMax4/2, Gain/1
  Divide/1 -> MinMax1/1  "max current"
  Divide1/1 -> MinMax2/1  "min current"
  Gain/1 -> MinMax3/2
  MinMax1/1 -> Divide2/2
  MinMax2/1 -> Divide3/2
  M/Iq/1 -> Divide2/1, Divide3/1
  Divide3/1 -> Saturation Dynamic7/2  "min torque"
  Torque2/1 -> Saturation Dynamic7/3
  Divide2/1 -> Subtract/2, Saturation Dynamic7/1  "max torque"
  Speed Limiting/1 -> Subtract/1, Subtract1/1
  Saturation Dynamic7/1 -> Subtract1/2
  Subtract/1 -> [M_max_upper_effective_r1538], "[r1538] Upper effective torque limit"/1
  Subtract1/1 -> [M_max_lower_effective_r1539], "[r1539] Lower effective torque limit"/1
  MinMax3/1 -> MinMax2/2
  Iq stall calculation/1 -> MinMax3/1
  MinMax4/1 -> MinMax1/2
  Iq stall calculation1/1 -> MinMax4/1
  Add4/1 -> Relational Operator1/2, Saturation Dynamic8/2
  1st order LPF1/1(Signal Out) -> "[r1516] Supplementary torque and acceleration torque "/1, Add4/1
  Gain3/1 -> Saturation Dynamic9/2, Relational Operator/2
  Saturation Dynamic9/1 -> Add4/2, Relational Operator/1, "[r1508] Torque setpoint before supplementary torque"/1
  [Torque_Limit_Lower_r1527] -> Saturation Dynamic10/2
  Saturation Dynamic11/1 -> Saturation Dynamic9/3, Saturation Dynamic8/3
  [M_max_upper_effective_r1538] -> Saturation Dynamic10/1
  [M_max_lower_effective_r1539] -> Saturation Dynamic10/3
  Torque3/1 -> Saturation Dynamic11/3
  Saturation Dynamic10/1 -> Saturation Dynamic11/2
  [Torque_Limit_Upper_r1526] -> MinMax5/2
  [M_max_upper_effective_r1538] -> Saturation Dynamic12/1, MinMax5/1
  Saturation Dynamic12/1 -> Saturation Dynamic8/1, Saturation Dynamic9/1, Saturation Dynamic11/1
  MinMax5/1 -> Saturation Dynamic12/2
  [M_max_lower_effective_r1539] -> Saturation Dynamic12/3
  Relational Operator/1 -> Logical Operator/2
  Relational Operator1/1 -> Logical Operator/1
  Logical Operator/1 -> [Torque_Limit_Reached_r1407_7]
  [Torque_Limit_Reached_r1407_7] -> Delay/1
  Product6/1 -> Product5/3
  Accelerating torque smoothing time constant/1 -> ms->s1/1
  ms->s1/1 -> 1st order LPF1/2(Time Constant)
  Gain4/1 -> 1st order LPF1/1(Signal)
  Delay/1 -> Logical Operator1/1
  Add1/1 -> Saturation Dynamic/2  "Speed setpoint from  [6030] speed setpoint, droop"
  "[r1170] n_ctrl setp sum (Speed setpoint after the RFG)"/1 -> Interpolator/1
  "[6050] Kp_n-/Tn_n adaptation NOTE: THE PARAMETERS USED CAUSE FIXED GAINS"/1(Kp_n_adapt) -> Gain1/1, "[r1468] Speed Controller P-gain effective"/1
  "[p21501] Droop Parameter from PLC"/1 -> Product1/2
  Logical Operator1/1 -> Product6/1
  Enable Speed Controller/1 -> Product4/3, Product6/2
  Gain1/1 -> [Kp_n_adapt]
  Gain6/1 -> [Tn_n_adapt]
  Discrete FIR Filter1/1 -> Discrete Derivative/1

== system DemonstratorSimscape/EM System/Drives/Simple Drive Model/Pwr Limits (R)/Limits ==
  TrqIn (Nm) : Inport
  MotSpd (rpm) : Inport  Port=2
  Abs : Abs
  Divide : Product  Inputs=*/
  Mux : Mux  Inputs=2
  Mux1 : Mux  Inputs=2
  Product : Product
  Pwr : Scope  Commented=on  NumInputPorts=2
  PwrLim : Saturate  UpperLimit=VSD.PwrMax*1e3  LowerLimit=-VSD.PwrMax*1e3
  Switch : Switch  Criteria=u2 > Threshold  Threshold=10
  TrqLim : Saturate  UpperLimit=VSD.TrqMax  LowerLimit=VSD.TrqMin
  rad/s : Gain  Gain=pi/30
  TrqSat (Nm) : Outport
  wires:
  Divide/1 -> Switch/1
  Mux1/1 -> Pwr/2
  Mux/1 -> Pwr/1
  MotSpd (rpm)/1 -> rad/s/1, Abs/1
  Switch/1 -> Mux1/2, TrqLim/1
  PwrLim/1 -> Divide/1, Mux/2
  Abs/1 -> Switch/2
  rad/s/1 -> Product/2, Divide/2
  Product/1 -> PwrLim/1, Mux/1
  TrqIn (Nm)/1 -> Product/1, Switch/3, Mux1/1
  TrqLim/1 -> TrqSat (Nm)/1

== system DemonstratorSimscape/EM System/Drives/Simple Drive Model/Pwr Limits (R)/No Limits ==
  TrqIn (Nm) : Inport
  MotSpd (rpm) : Inport  Port=2
  TrqSat (Nm) : Outport
  wires:
  TrqIn (Nm)/1 -> TrqSat (Nm)/1

== system DemonstratorSimscape/EM System/Drives/Simple Drive Model/Spd Limits1/DerSatInt ==
  SpdIn : Inport
  Discrete Derivative : simulink/Discrete/Discrete Derivative  gainval=1.0  ICPrevScaledInput=0.0  OutMin=[]  OutMax=[]  OutDataType=fixdt(1, 16)  OutScaling=2^-10  DoSatur=off
  Discrete-Time Integrator : DiscreteIntegrator  IntegratorMethod=Integration: Backward Euler  SampleTime=-1  ICPrevOutput=DiscIntNeverNeededParam  ICPrevScaledInput=DiscIntNeverNeededParam
  Saturation : Saturate  UpperLimit=VSD.SpdRateLimPos  LowerLimit=VSD.SpdRateLimNeg
  SpdLim : Outport
  RateSat : Outport  Port=2
  Rate : Outport  Port=3
  wires:
  Discrete-Time Integrator/1 -> SpdLim/1
  SpdIn/1 -> Discrete Derivative/1
  Discrete Derivative/1 -> Saturation/1, Rate/1
  Saturation/1 -> Discrete-Time Integrator/1, RateSat/1

== system DemonstratorSimscape/EM System/Drives/Simple Drive Model/Spd Limits1/No Rate Limits ==
  SpdIn : Inport
  SpdLim : Outport
  wires:
  SpdIn/1 -> SpdLim/1

== system DemonstratorSimscape/EM System/Drives/Simple Drive Model/Spd Limits1/Rate Limiter ==
  SpdIn : Inport
  Add : Sum  Inputs=+-
  Gain : Gain  Gain=1/0.01
  Unit Delay : UnitDelay  SampleTime=-1  HasFrameUpgradeWarning=on
  VSD SpdRef Rate Limiter2 : RateLimiter  RisingSlewLimit=VSD.SpdRateLimPos  FallingSlewLimit=VSD.SpdRateLimNeg  SampleTimeMode=inherited
  SpdLim : Outport
  RateSat : Outport  Port=2
  wires:
  Gain/1 -> RateSat/1
  SpdIn/1 -> VSD SpdRef Rate Limiter2/1, Add/1
  Add/1 -> Gain/1
  Unit Delay/1 -> Add/2
  VSD SpdRef Rate Limiter2/1 -> Unit Delay/1, SpdLim/1

== system DemonstratorSimscape/EM System/Drives/Simple Drive Model1/Pwr Limits (L)/Limits ==
  TrqIn (Nm) : Inport
  MotSpd (rpm) : Inport  Port=2
  Abs : Abs
  Divide : Product  Inputs=*/
  Mux : Mux  Inputs=2
  Mux1 : Mux  Inputs=3
  Product : Product
  Pwr : Scope  Commented=on  NumInputPorts=2
  PwrLim : Saturate  UpperLimit=VSD.PwrMax*1e3  LowerLimit=-VSD.PwrMax*1e3
  Switch : Switch  Criteria=u2 > Threshold  Threshold=10
  TrqLim : Saturate  UpperLimit=VSD.TrqMax  LowerLimit=VSD.TrqMin
  rad/s : Gain  Gain=pi/30
  TrqSat (Nm) : Outport
  wires:
  TrqLim/1 -> TrqSat (Nm)/1, Mux1/3
  Divide/1 -> Switch/1
  Mux1/1 -> Pwr/2
  Mux/1 -> Pwr/1
  MotSpd (rpm)/1 -> rad/s/1, Abs/1
  Switch/1 -> TrqLim/1, Mux1/2
  PwrLim/1 -> Divide/1, Mux/2
  Abs/1 -> Switch/2
  rad/s/1 -> Product/2, Divide/2
  Product/1 -> PwrLim/1, Mux/1
  TrqIn (Nm)/1 -> Product/1, Switch/3, Mux1/1

== system DemonstratorSimscape/EM System/Drives/Simple Drive Model1/Pwr Limits (L)/No Limits ==
  TrqIn (Nm) : Inport
  MotSpd (rpm) : Inport  Port=2
  TrqSat (Nm) : Outport
  wires:
  TrqIn (Nm)/1 -> TrqSat (Nm)/1

== system DemonstratorSimscape/EM System/Drives/Simple Drive Model1/Pwr Limits (R)/Limits ==
  TrqIn (Nm) : Inport
  MotSpd (rpm) : Inport  Port=2
  Abs : Abs
  Divide : Product  Inputs=*/
  Mux : Mux  Inputs=2
  Mux1 : Mux  Inputs=2
  Product : Product
  Pwr : Scope  Commented=on  NumInputPorts=2
  PwrLim : Saturate  UpperLimit=VSD.PwrMax*1e3  LowerLimit=-VSD.PwrMax*1e3
  Switch : Switch  Criteria=u2 > Threshold  Threshold=10
  TrqLim : Saturate  UpperLimit=VSD.TrqMax  LowerLimit=VSD.TrqMin
  rad/s : Gain  Gain=pi/30
  TrqSat (Nm) : Outport
  wires:
  TrqLim/1 -> TrqSat (Nm)/1
  TrqIn (Nm)/1 -> Mux1/1, Switch/3, Product/1
  Product/1 -> Mux/1, PwrLim/1
  rad/s/1 -> Divide/2, Product/2
  Abs/1 -> Switch/2
  PwrLim/1 -> Mux/2, Divide/1
  Switch/1 -> TrqLim/1, Mux1/2
  MotSpd (rpm)/1 -> Abs/1, rad/s/1
  Mux/1 -> Pwr/1
  Mux1/1 -> Pwr/2
  Divide/1 -> Switch/1

== system DemonstratorSimscape/EM System/Drives/Simple Drive Model1/Pwr Limits (R)/No Limits ==
  TrqIn (Nm) : Inport
  MotSpd (rpm) : Inport  Port=2
  TrqSat (Nm) : Outport
  wires:
  TrqIn (Nm)/1 -> TrqSat (Nm)/1

== system DemonstratorSimscape/EM System/Drives/Simple Drive Model1/Spd Limits/DerSatInt ==
  SpdIn : Inport
  Discrete Derivative : simulink/Discrete/Discrete Derivative  gainval=1.0  ICPrevScaledInput=0.0  OutMin=[]  OutMax=[]  OutDataType=fixdt(1, 16)  OutScaling=2^-10  DoSatur=off
  Discrete-Time Integrator : DiscreteIntegrator  IntegratorMethod=Integration: Backward Euler  SampleTime=-1  ICPrevOutput=DiscIntNeverNeededParam  ICPrevScaledInput=DiscIntNeverNeededParam
  Saturation : Saturate  UpperLimit=VSD.SpdRateLimPos  LowerLimit=VSD.SpdRateLimNeg
  SpdLim : Outport
  RateSat : Outport  Port=2
  Rate : Outport  Port=3
  wires:
  Discrete-Time Integrator/1 -> SpdLim/1
  SpdIn/1 -> Discrete Derivative/1
  Discrete Derivative/1 -> Saturation/1, Rate/1
  Saturation/1 -> Discrete-Time Integrator/1, RateSat/1

== system DemonstratorSimscape/EM System/Drives/Simple Drive Model1/Spd Limits/No Rate Limits ==
  SpdIn : Inport
  SpdLim : Outport
  wires:
  SpdIn/1 -> SpdLim/1

== system DemonstratorSimscape/EM System/Drives/Simple Drive Model1/Spd Limits/Rate Limiter ==
  SpdIn : Inport
  Add : Sum  Inputs=+-
  Gain : Gain  Gain=1/0.01
  Unit Delay : UnitDelay  SampleTime=-1  HasFrameUpgradeWarning=on
  VSD SpdRef Rate Limiter2 : RateLimiter  RisingSlewLimit=VSD.SpdRateLimPos  FallingSlewLimit=VSD.SpdRateLimNeg  SampleTimeMode=inherited
  SpdLim : Outport
  RateSat : Outport  Port=2
  wires:
  Gain/1 -> RateSat/1
  SpdIn/1 -> VSD SpdRef Rate Limiter2/1, Add/1
  Add/1 -> Gain/1
  Unit Delay/1 -> Add/2
  VSD SpdRef Rate Limiter2/1 -> Unit Delay/1, SpdLim/1

== system DemonstratorSimscape/EM System/Drives/Simple Drive Model1/Spd Limits1/DerSatInt ==
  SpdIn : Inport
  Discrete Derivative : simulink/Discrete/Discrete Derivative  gainval=1.0  ICPrevScaledInput=0.0  OutMin=[]  OutMax=[]  OutDataType=fixdt(1, 16)  OutScaling=2^-10  DoSatur=off
  Discrete-Time Integrator : DiscreteIntegrator  IntegratorMethod=Integration: Backward Euler  SampleTime=-1  ICPrevOutput=DiscIntNeverNeededParam  ICPrevScaledInput=DiscIntNeverNeededParam
  Saturation : Saturate  UpperLimit=VSD.SpdRateLimPos  LowerLimit=VSD.SpdRateLimNeg
  SpdLim : Outport
  RateSat : Outport  Port=2
  Rate : Outport  Port=3
  wires:
  Saturation/1 -> RateSat/1, Discrete-Time Integrator/1
  Discrete Derivative/1 -> Rate/1, Saturation/1
  SpdIn/1 -> Discrete Derivative/1
  Discrete-Time Integrator/1 -> SpdLim/1

== system DemonstratorSimscape/EM System/Drives/Simple Drive Model1/Spd Limits1/No Rate Limits ==
  SpdIn : Inport
  SpdLim : Outport
  wires:
  SpdIn/1 -> SpdLim/1

== system DemonstratorSimscape/EM System/Drives/Simple Drive Model1/Spd Limits1/Rate Limiter ==
  SpdIn : Inport
  Add : Sum  Inputs=+-
  Gain : Gain  Gain=1/0.01
  Unit Delay : UnitDelay  SampleTime=-1  HasFrameUpgradeWarning=on
  VSD SpdRef Rate Limiter2 : RateLimiter  RisingSlewLimit=VSD.SpdRateLimPos  FallingSlewLimit=VSD.SpdRateLimNeg  SampleTimeMode=inherited
  SpdLim : Outport
  RateSat : Outport  Port=2
  wires:
  VSD SpdRef Rate Limiter2/1 -> SpdLim/1, Unit Delay/1
  Unit Delay/1 -> Add/2
  Add/1 -> Gain/1
  SpdIn/1 -> Add/1, VSD SpdRef Rate Limiter2/1
  Gain/1 -> RateSat/1

== system DemonstratorSimscape/Transmission System/Anchor and Load/Load/DOUBLE/Cable_Left ==
  In1 : Inport
  Gain : Gain  Gain=0.5
  Simulink-PS Converter1 : nesl_utility/Simulink-PS Converter  PhysicalDomain=network_engine_domain  SubClassName=ps_input  LeftPortType=input  RightPortType=output  PseudoPeriodic=off  Frequencies=[]  NoiseDistribution=none  NoiseParameters=[]  Unit=kg  AffineConversion=on  FilteringAndDerivatives=zero  SimscapeFilterOrder=2  InputFilterTimeConstant=0.001  UdotUserProvided=0
  cable Variable Mass1 : sm_lib/Body Elements/Variable Mass/General Variable Mass  VariableInertiaType=PointMass  MassType=TimeVarying  Mass=1  MassUnits=kg  CenterOfMassType=Constant  CenterOfMass=[0 0 0]  CenterOfMassUnits=m  InertiaMatrixType=TimeVarying  MomentsOfInertia=[1 1 1]  MomentsOfInertiaUnits=kg*m^2  ProductsOfInertia=[0 0 0]  ProductsOfInertiaUnits=kg*m^2  GraphicType=None  MarkerShape=Sphere  MarkerSize=10  GraphicVisPropType=SimpleVisualProperties  GraphicDiffuseColor=[0.5 0.5 0.5]  GraphicSpecularColor=[0.5 0.5 0.5 1.0]  GraphicAmbientColor=[0.15 0.15 0.15 1.0]  GraphicEmissiveColor=[0.0 0.0 0.0 1.0]  GraphicShininess=75  GraphicOpacity=1.0
      settings: SourceProductBaseCode=MS
  Conn1 : PMIOPort  Side=Right
  wires:
  Gain/1 -> Simulink-PS Converter1/1
  In1/1 -> Gain/1
  connections:
  Conn1/RConn1 -- cable Variable Mass1/RConn1
  Simulink-PS Converter1/RConn1 -- cable Variable Mass1/LConn1

== system DemonstratorSimscape/Transmission System/Anchor and Load/Load/DOUBLE/Cable_Right ==
  In1 : Inport
  Gain1 : Gain  Gain=0.5
  Simulink-PS Converter2 : nesl_utility/Simulink-PS Converter  PhysicalDomain=network_engine_domain  SubClassName=ps_input  LeftPortType=input  RightPortType=output  PseudoPeriodic=off  Frequencies=[]  NoiseDistribution=none  NoiseParameters=[]  Unit=kg  AffineConversion=on  FilteringAndDerivatives=zero  SimscapeFilterOrder=2  InputFilterTimeConstant=0.001  UdotUserProvided=0
  cable Variable Mass2 : sm_lib/Body Elements/Variable Mass/General Variable Mass  VariableInertiaType=PointMass  MassType=TimeVarying  Mass=1  MassUnits=kg  CenterOfMassType=Constant  CenterOfMass=[0 0 0]  CenterOfMassUnits=m  InertiaMatrixType=TimeVarying  MomentsOfInertia=[1 1 1]  MomentsOfInertiaUnits=kg*m^2  ProductsOfInertia=[0 0 0]  ProductsOfInertiaUnits=kg*m^2  GraphicType=None  MarkerShape=Sphere  MarkerSize=10  GraphicVisPropType=SimpleVisualProperties  GraphicDiffuseColor=[0.5 0.5 0.5]  GraphicSpecularColor=[0.5 0.5 0.5 1.0]  GraphicAmbientColor=[0.15 0.15 0.15 1.0]  GraphicEmissiveColor=[0.0 0.0 0.0 1.0]  GraphicShininess=75  GraphicOpacity=1.0
      settings: SourceProductBaseCode=MS
  Conn1 : PMIOPort  Side=Right
  wires:
  Gain1/1 -> Simulink-PS Converter2/1
  In1/1 -> Gain1/1
  connections:
  Simulink-PS Converter2/RConn1 -- cable Variable Mass2/LConn1
  cable Variable Mass2/RConn1 -- Conn1/RConn1
